simulink model "kaiguangai1108"  (R2016b)
settings: Solver=ode4  StartTime=0.0  StopTime=inf  FixedStep=0.002  RelTol=1e-3  EnableMultiTasking=on
libraries: slrtlib x5
(part 2 of 6)

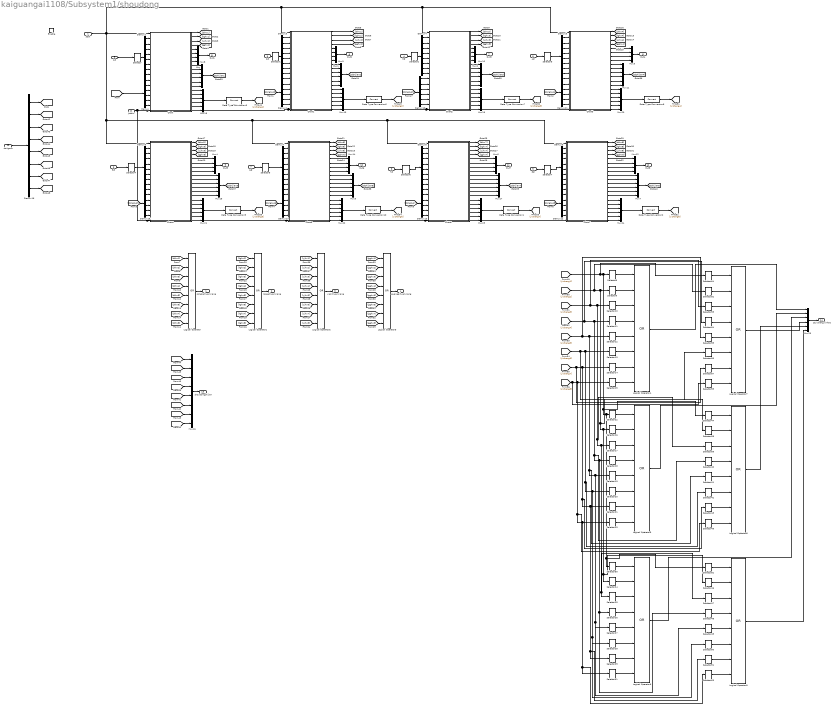
== system kaiguangai1108/Subsystem1/shoudong ==
  start : Inport
  1# : Inport  Port=2
  2# : Inport  Port=3
  3# : Inport  Port=4
  4# : Inport  Port=5
  5# : Inport  Port=6
  6# : Inport  Port=7
  7# : Inport  Port=8
  8# : Inport  Port=9
  dongzuo : Inport  Port=10
  jieshu : Inport  Port=11
  Enable : EnablePort
  Chart : Stateflow chart  TreatAsAtomicUnit=on
  Chart1 : Stateflow chart  TreatAsAtomicUnit=on
  Chart2 : Stateflow chart  TreatAsAtomicUnit=on
  Chart3 : Stateflow chart  TreatAsAtomicUnit=on
  Chart4 : Stateflow chart  TreatAsAtomicUnit=on
  Chart5 : Stateflow chart  TreatAsAtomicUnit=on
  Chart6 : Stateflow chart  TreatAsAtomicUnit=on
  Chart7 : Stateflow chart  TreatAsAtomicUnit=on
  Data Type Conversion{1..2,5..10} (8 alike) : DataTypeConversion
  Demux{,1,10..15} (8 alike) : Demux  Outputs=6
  Demux{2..9,16} (9 alike) : Demux  Outputs=8
  Logical Operator{,1..9} (10 alike) : Logic  Operator=OR  Inputs=8  AllPortsSameDT=off  OutDataTypeStr=boolean
  Mux{,1..4,6,12,14} (8 alike) : Mux
  Mux{5,7..11,13,15,17..25} (17 alike) : Mux  Inputs=6
  Mux16 : Mux  Inputs=8
  Selector{,1..7} (8 alike) : Selector  IndexOptions=Index vector (dialog)  Indices=[1:4 7:10]  OutputSizes=1
  Selector{8..15} (8 alike) : Selector  IndexOptions=Index vector (dialog)  Indices=[1]  OutputSizes=1
  Selector{16..23} (8 alike) : Selector  IndexOptions=Index vector (dialog)  Indices=[2]  OutputSizes=1
  Selector{24..31} (8 alike) : Selector  IndexOptions=Index vector (dialog)  Indices=[3]  OutputSizes=1
  Selector{32..37,54..55} (8 alike) : Selector  IndexOptions=Index vector (dialog)  Indices=[4]  OutputSizes=1
  Selector{38..45} (8 alike) : Selector  IndexOptions=Index vector (dialog)  Indices=[5]  OutputSizes=1
  Selector{46..53} (8 alike) : Selector  IndexOptions=Index vector (dialog)  Indices=[6]  OutputSizes=1
  songkaihuanxiang : Outport
  kaigaihuanxiang : Outport  Port=2
  yajinhuanxiang : Outport  Port=3
  guangaihuanxiang : Outport  Port=4
  Out1 : Outport  Port=5
  Out2 : Outport  Port=6
  Out3 : Outport  Port=7
  Out4 : Outport  Port=8
  Out5 : Outport  Port=9
  Out6 : Outport  Port=10
  Out7 : Outport  Port=11
  Out8 : Outport  Port=12
  shoudongshijian : Outport  Port=13
  sdyichangxinhao : Outport  Port=14
  wires:
  Demux14/2 -> Chart5/11(kaigai)
  Demux14/3 -> Chart5/12(suoding)
  Demux14/1 -> Chart5/10(songkai)
  Demux14/4 -> Chart5/13(jiesuo)
  Demux14/5 -> Chart5/14(guangai)
  Demux14/6 -> Chart5/15(yajin)
  Demux11/4 -> Chart3/13(jiesuo)
  Demux11/5 -> Chart3/14(guangai)
  Demux11/6 -> Chart3/15(yajin)
  Demux13/1 -> Chart6/10(songkai)
  Demux13/2 -> Chart6/11(kaigai)
  Demux13/3 -> Chart6/12(suoding)
  Demux13/4 -> Chart6/13(jiesuo)
  Demux13/5 -> Chart6/14(guangai)
  Demux13/6 -> Chart6/15(yajin)
  Demux9/5 -> Chart7/6(sddw)
  Demux9/6 -> Chart7/7(jsdw)
  Demux9/4 -> Chart7/5(ggdw2)
  Demux9/1 -> Chart7/2(kgdw1)
  Demux9/3 -> Chart7/4(ggdw1)
  Demux9/2 -> Chart7/3(kgdw2)
  Demux9/7 -> Chart7/8(yjdw)
  8#/1 -> Selector7/1
  Demux9/8 -> Chart7/9(skdw)
  Demux11/1 -> Chart3/10(songkai)
  Demux11/2 -> Chart3/11(kaigai)
  Demux11/3 -> Chart3/12(suoding)
  Demux1/1 -> Chart1/10(songkai)
  Demux1/3 -> Chart1/12(suoding)
  Demux1/2 -> Chart1/11(kaigai)
  Demux1/4 -> Chart1/13(jiesuo)
  Demux1/5 -> Chart1/14(guangai)
  Demux1/6 -> Chart1/15(yajin)
  Demux10/1 -> Chart2/10(songkai)
  Demux10/2 -> Chart2/11(kaigai)
  Demux10/4 -> Chart2/13(jiesuo)
  Demux10/5 -> Chart2/14(guangai)
  Demux10/6 -> Chart2/15(yajin)
  Demux10/3 -> Chart2/12(suoding)
  Demux6/1 -> Chart4/2(kgdw1)
  Demux6/2 -> Chart4/3(kgdw2)
  Demux6/3 -> Chart4/4(ggdw1)
  Demux6/4 -> Chart4/5(ggdw2)
  Demux6/5 -> Chart4/6(sddw)
  Demux6/6 -> Chart4/7(jsdw)
  Demux6/7 -> Chart4/8(yjdw)
  Demux6/8 -> Chart4/9(skdw)
  Demux2/3 -> Chart/4(ggdw1)
  Demux8/3 -> Chart6/4(ggdw1)
  Demux8/4 -> Chart6/5(ggdw2)
  Demux8/1 -> Chart6/2(kgdw1)
  Demux8/2 -> Chart6/3(kgdw2)
  Demux8/5 -> Chart6/6(sddw)
  Demux12/1 -> Chart7/10(songkai)
  Demux12/2 -> Chart7/11(kaigai)
  Demux8/8 -> Chart6/9(skdw)
  Demux8/7 -> Chart6/8(yjdw)
  Demux12/3 -> Chart7/12(suoding)
  Demux8/6 -> Chart6/7(jsdw)
  Demux12/6 -> Chart7/15(yajin)
  Demux12/5 -> Chart7/14(guangai)
  Demux12/4 -> Chart7/13(jiesuo)
  Demux15/2 -> Chart4/11(kaigai)
  Demux15/1 -> Chart4/10(songkai)
  Demux5/4 -> Chart3/5(ggdw2)
  Demux5/6 -> Chart3/7(jsdw)
  Demux5/3 -> Chart3/4(ggdw1)
  Demux5/7 -> Chart3/8(yjdw)
  Demux5/5 -> Chart3/6(sddw)
  Demux5/2 -> Chart3/3(kgdw2)
  Demux15/3 -> Chart4/12(suoding)
  Demux5/1 -> Chart3/2(kgdw1)
  4#/1 -> Selector3/1
  Demux5/8 -> Chart3/9(skdw)
  Demux2/7 -> Chart/8(yjdw)
  Demux15/4 -> Chart4/13(jiesuo)
  Demux15/5 -> Chart4/14(guangai)
  Demux15/6 -> Chart4/15(yajin)
  Demux/4 -> Chart/13(jiesuo)
  Demux/5 -> Chart/14(guangai)
  Demux/6 -> Chart/15(yajin)
  Demux2/2 -> Chart/3(kgdw2)
  Demux2/1 -> Chart/2(kgdw1)
  Demux4/2 -> Chart2/3(kgdw2)
  Demux4/3 -> Chart2/4(ggdw1)
  Demux4/4 -> Chart2/5(ggdw2)
  Demux4/5 -> Chart2/6(sddw)
  Demux4/1 -> Chart2/2(kgdw1)
  Demux4/7 -> Chart2/8(yjdw)
  Demux4/6 -> Chart2/7(jsdw)
  Demux4/8 -> Chart2/9(skdw)
  Demux2/4 -> Chart/5(ggdw2)
  Demux2/5 -> Chart/6(sddw)
  Demux2/6 -> Chart/7(jsdw)
  Demux3/2 -> Chart1/3(kgdw2)
  Demux3/3 -> Chart1/4(ggdw1)
  Demux3/4 -> Chart1/5(ggdw2)
  Demux3/6 -> Chart1/7(jsdw)
  Demux3/7 -> Chart1/8(yjdw)
  Demux3/8 -> Chart1/9(skdw)
  Demux2/8 -> Chart/9(skdw)
  Demux3/5 -> Chart1/6(sddw)
  Demux3/1 -> Chart1/2(kgdw1)
  Demux/1 -> Chart/10(songkai)
  Demux/2 -> Chart/11(kaigai)
  Demux/3 -> Chart/12(suoding)
  Demux7/2 -> Chart5/3(kgdw2)
  Demux7/5 -> Chart5/6(sddw)
  Demux7/3 -> Chart5/4(ggdw1)
  Demux7/1 -> Chart5/2(kgdw1)
  Demux7/8 -> Chart5/9(skdw)
  Demux7/4 -> Chart5/5(ggdw2)
  6#/1 -> Selector5/1
  Demux7/6 -> Chart5/7(jsdw)
  Demux7/7 -> Chart5/8(yjdw)
  5#/1 -> Selector4/1
  7#/1 -> Selector6/1
  [dongzuo2] -> Demux1/1
  [dongzuo3] -> Demux10/1
  [dongzuo4] -> Demux11/1
  [dongzuo5] -> Demux15/1
  [dongzuo6] -> Demux14/1
  [dongzuo7] -> Demux13/1
  [dongzuo8] -> Demux12/1
  Chart/1(skhx) -> [skhx1]
  Chart/2(kghx) -> [kghx1]
  Chart/3(yjhx) -> [yjhx1]
  Chart/4(gghx) -> [gghx1]
  Chart1/1(skhx) -> [skhx2]
  Chart1/2(kghx) -> [kghx2]
  Chart1/3(yjhx) -> [yjhx2]
  Chart1/4(gghx) -> [gghx2]
  Chart2/1(skhx) -> [skhx3]
  Chart2/2(kghx) -> [kghx3]
  Chart2/3(yjhx) -> [yjhx3]
  Chart2/4(gghx) -> [gghx3]
  Chart3/1(skhx) -> [skhx4]
  Chart3/2(kghx) -> [kghx4]
  Chart3/3(yjhx) -> [yjhx4]
  Chart3/4(gghx) -> [gghx4]
  Chart4/1(skhx) -> [skhx5]
  Chart5/1(skhx) -> [skhx6]
  Chart5/2(kghx) -> [kghx6]
  Chart5/4(gghx) -> [gghx6]
  Chart7/1(skhx) -> [skhx8]
  Chart7/2(kghx) -> [kghx8]
  Chart7/3(yjhx) -> [yjhx8]
  Chart7/4(gghx) -> [gghx8]
  [skhx1] -> Logical Operator/1
  [skhx2] -> Logical Operator/2
  [skhx3] -> Logical Operator/3
  [skhx4] -> Logical Operator/4
  [skhx5] -> Logical Operator/5
  [skhx6] -> Logical Operator/6
  [skhx7] -> Logical Operator/7
  [skhx8] -> Logical Operator/8
  Logical Operator/1 -> songkaihuanxiang/1
  [kghx1] -> Logical Operator1/1
  [kghx2] -> Logical Operator1/2
  [kghx3] -> Logical Operator1/3
  [kghx4] -> Logical Operator1/4
  [kghx5] -> Logical Operator1/5
  [kghx6] -> Logical Operator1/6
  [kghx7] -> Logical Operator1/7
  [kghx8] -> Logical Operator1/8
  Logical Operator1/1 -> kaigaihuanxiang/1
  [yjhx1] -> Logical Operator2/1
  [yjhx2] -> Logical Operator2/2
  [yjhx3] -> Logical Operator2/3
  [yjhx4] -> Logical Operator2/4
  [yjhx5] -> Logical Operator2/5
  [yjhx6] -> Logical Operator2/6
  [yjhx7] -> Logical Operator2/7
  [yjhx8] -> Logical Operator2/8
  Logical Operator2/1 -> yajinhuanxiang/1
  [gghx1] -> Logical Operator3/1
  [gghx2] -> Logical Operator3/2
  [gghx3] -> Logical Operator3/3
  [gghx4] -> Logical Operator3/4
  [gghx5] -> Logical Operator3/5
  [gghx6] -> Logical Operator3/6
  [gghx7] -> Logical Operator3/7
  [gghx8] -> Logical Operator3/8
  Logical Operator3/1 -> guangaihuanxiang/1
  Chart/5(kgzhiling1) -> Mux/1
  Chart/6(kgzhiling2) -> Mux/2
  Chart/7(ggzhiling1) -> Mux/3
  Chart/8(ggzhiling2) -> Mux/4
  Chart1/5(kgzhiling1) -> Mux1/1
  Chart1/6(kgzhiling2) -> Mux1/2
  Chart1/7(ggzhiling1) -> Mux1/3
  Chart1/8(ggzhiling2) -> Mux1/4
  Chart2/5(kgzhiling1) -> Mux2/1
  Chart2/6(kgzhiling2) -> Mux2/2
  Chart2/7(ggzhiling1) -> Mux2/3
  Chart2/8(ggzhiling2) -> Mux2/4
  Mux/1 -> Out1/1
  Mux1/1 -> Out2/1
  Mux2/1 -> Out3/1
  Mux4/1 -> Out5/1
  Mux14/1 -> Out6/1
  Chart/9(skt) -> Mux8/1
  Chart/10(kgt) -> Mux8/2
  Chart/11(sdt) -> Mux8/3
  Chart/12(jst) -> Mux8/4
  Chart/13(ggt) -> Mux8/5
  Chart/14(yjt) -> Mux8/6
  Chart1/9(skt) -> Mux9/1
  Chart1/10(kgt) -> Mux9/2
  Chart1/11(sdt) -> Mux9/3
  Chart1/12(jst) -> Mux9/4
  Chart1/13(ggt) -> Mux9/5
  Chart1/14(yjt) -> Mux9/6
  Mux8/1 -> [sdshijian1]
  Mux9/1 -> [sdshijian2]
  Mux17/1 -> [sdshijian7]
  [sdshijian1] -> Mux16/1
  [sdshijian2] -> Mux16/2
  [sdshijian3] -> Mux16/3
  [sdshijian4] -> Mux16/4
  [sdshijian5] -> Mux16/5
  [sdshijian6] -> Mux16/6
  [sdshijian7] -> Mux16/7
  [sdshijian8] -> Mux16/8
  Mux16/1 -> shoudongshijian/1
  Selector/1 -> Demux2/1
  1#/1 -> Selector/1
  2#/1 -> Selector1/1
  Selector1/1 -> Demux3/1
  Selector2/1 -> Demux4/1
  3#/1 -> Selector2/1
  Selector3/1 -> Demux5/1
  Selector4/1 -> Demux6/1
  Selector5/1 -> Demux7/1
  Selector6/1 -> Demux8/1
  Selector7/1 -> Demux9/1
  jieshu/1 -> Chart7/16(jieshu), Chart6/16(jieshu), Chart5/16(jieshu), Chart4/16(jieshu), Chart3/16(jieshu), Chart2/16(jieshu), Chart1/16(jieshu), Chart/16(jieshu)
  Demux16/1 -> [dongzuo1]
  [dongzuo1] -> Demux/1
  Demux16/2 -> [dongzuo2]
  Demux16/3 -> [dongzuo3]
  Demux16/4 -> [dongzuo4]
  Demux16/5 -> [dongzuo5]
  Demux16/6 -> [dongzuo6]
  Demux16/7 -> [dongzuo7]
  Demux16/8 -> [dongzuo8]
  dongzuo/1 -> Demux16/1
  Chart2/14(yjt) -> Mux10/6
  Chart2/13(ggt) -> Mux10/5
  Chart2/12(jst) -> Mux10/4
  Chart2/11(sdt) -> Mux10/3
  Chart2/10(kgt) -> Mux10/2
  Chart2/9(skt) -> Mux10/1
  Mux10/1 -> [sdshijian3]
  Chart3/8(ggzhiling2) -> Mux3/4
  Chart3/7(ggzhiling1) -> Mux3/3
  Chart3/6(kgzhiling2) -> Mux3/2
  Chart3/5(kgzhiling1) -> Mux3/1
  Mux3/1 -> Out4/1
  Chart3/9(skt) -> Mux11/1
  Chart3/10(kgt) -> Mux11/2
  Chart3/11(sdt) -> Mux11/3
  Chart3/12(jst) -> Mux11/4
  Chart3/13(ggt) -> Mux11/5
  Chart3/14(yjt) -> Mux11/6
  Mux11/1 -> [sdshijian4]
  Chart4/2(kghx) -> [kghx5]
  Chart4/3(yjhx) -> [yjhx5]
  Chart4/4(gghx) -> [gghx5]
  Chart4/5(kgzhiling1) -> Mux4/1
  Chart4/6(kgzhiling2) -> Mux4/2
  Chart4/7(ggzhiling1) -> Mux4/3
  Chart4/8(ggzhiling2) -> Mux4/4
  Chart4/9(skt) -> Mux15/1
  Chart4/10(kgt) -> Mux15/2
  Chart4/11(sdt) -> Mux15/3
  Chart4/12(jst) -> Mux15/4
  Chart4/13(ggt) -> Mux15/5
  Chart4/14(yjt) -> Mux15/6
  Mux15/1 -> [sdshijian5]
  Chart5/3(yjhx) -> [yjhx6]
  Chart5/5(kgzhiling1) -> Mux14/1
  Chart5/6(kgzhiling2) -> Mux14/2
  Chart5/7(ggzhiling1) -> Mux14/3
  Chart5/8(ggzhiling2) -> Mux14/4
  Chart5/9(skt) -> Mux5/1
  Chart5/10(kgt) -> Mux5/2
  Chart5/11(sdt) -> Mux5/3
  Chart5/12(jst) -> Mux5/4
  Chart5/13(ggt) -> Mux5/5
  Chart5/14(yjt) -> Mux5/6
  Mux5/1 -> [sdshijian6]
  Chart6/1(skhx) -> [skhx7]
  Chart6/2(kghx) -> [kghx7]
  Chart6/3(yjhx) -> [yjhx7]
  Chart6/4(gghx) -> [gghx7]
  Chart6/8(ggzhiling2) -> Mux6/4
  Chart6/7(ggzhiling1) -> Mux6/3
  Chart6/6(kgzhiling2) -> Mux6/2
  Chart6/5(kgzhiling1) -> Mux6/1
  Mux6/1 -> Out7/1
  Chart6/10(kgt) -> Mux17/2
  Chart6/11(sdt) -> Mux17/3
  Chart6/12(jst) -> Mux17/4
  Chart6/13(ggt) -> Mux17/5
  Chart6/14(yjt) -> Mux17/6
  Chart6/9(skt) -> Mux17/1
  Mux7/1 -> [sdshijian8]
  Chart7/8(ggzhiling2) -> Mux12/4
  Chart7/7(ggzhiling1) -> Mux12/3
  Chart7/6(kgzhiling2) -> Mux12/2
  Chart7/5(kgzhiling1) -> Mux12/1
  Mux12/1 -> Out8/1
  Chart7/10(kgt) -> Mux7/2
  Chart7/11(sdt) -> Mux7/3
  Chart7/12(jst) -> Mux7/4
  Chart7/13(ggt) -> Mux7/5
  Chart7/14(yjt) -> Mux7/6
  Chart7/9(skt) -> Mux7/1
  Chart1/15(skyichang) -> Mux13/1
  Chart1/16(kgyichang) -> Mux13/2
  Chart1/17(sdyichang) -> Mux13/3
  Chart1/18(jsyichang) -> Mux13/4
  Chart1/19(ggyichang) -> Mux13/5
  Chart1/20(yjyichang) -> Mux13/6
  Chart/15(skyichang) -> Mux18/1
  Chart/16(kgyichang) -> Mux18/2
  Chart/17(sdyichang) -> Mux18/3
  Chart/18(jsyichang) -> Mux18/4
  Chart/19(ggyichang) -> Mux18/5
  Chart/20(yjyichang) -> Mux18/6
  Chart2/15(skyichang) -> Mux19/1
  Chart2/16(kgyichang) -> Mux19/2
  Chart2/17(sdyichang) -> Mux19/3
  Chart2/18(jsyichang) -> Mux19/4
  Chart2/19(ggyichang) -> Mux19/5
  Chart2/20(yjyichang) -> Mux19/6
  Chart3/15(skyichang) -> Mux20/1
  Chart3/16(kgyichang) -> Mux20/2
  Chart3/17(sdyichang) -> Mux20/3
  Chart3/18(jsyichang) -> Mux20/4
  Chart3/19(ggyichang) -> Mux20/5
  Chart3/20(yjyichang) -> Mux20/6
  Chart4/15(skyichang) -> Mux21/1
  Chart4/16(kgyichang) -> Mux21/2
  Chart4/17(sdyichang) -> Mux21/3
  Chart4/18(jsyichang) -> Mux21/4
  Chart4/19(ggyichang) -> Mux21/5
  Chart4/20(yjyichang) -> Mux21/6
  Chart5/15(skyichang) -> Mux22/1
  Chart5/16(kgyichang) -> Mux22/2
  Chart5/17(sdyichang) -> Mux22/3
  Chart5/18(jsyichang) -> Mux22/4
  Chart5/19(ggyichang) -> Mux22/5
  Chart5/20(yjyichang) -> Mux22/6
  Chart6/15(skyichang) -> Mux23/1
  Chart6/16(kgyichang) -> Mux23/2
  Chart6/17(sdyichang) -> Mux23/3
  Chart6/18(jsyichang) -> Mux23/4
  Chart6/19(ggyichang) -> Mux23/5
  Chart6/20(yjyichang) -> Mux23/6
  Chart7/15(skyichang) -> Mux24/1
  Chart7/16(kgyichang) -> Mux24/2
  Chart7/17(sdyichang) -> Mux24/3
  Chart7/18(jsyichang) -> Mux24/4
  Chart7/19(ggyichang) -> Mux24/5
  Chart7/20(yjyichang) -> Mux24/6
  Mux18/1 -> Data Type Conversion5/1
  Data Type Conversion5/1 -> [yichang1]
  Mux13/1 -> Data Type Conversion6/1
  Data Type Conversion6/1 -> [yichang2]
  Mux19/1 -> Data Type Conversion7/1
  Data Type Conversion7/1 -> [yichang3]
  Mux20/1 -> Data Type Conversion8/1
  Data Type Conversion8/1 -> [yichang4]
  Mux21/1 -> Data Type Conversion9/1
  Data Type Conversion9/1 -> [yichang5]
  Mux22/1 -> Data Type Conversion10/1
  Data Type Conversion10/1 -> [yichang6]
  Mux23/1 -> Data Type Conversion1/1
  Data Type Conversion1/1 -> [yichang7]
  Mux24/1 -> Data Type Conversion2/1
  Data Type Conversion2/1 -> [yichang8]
  start/1 -> Chart/1(start), Chart4/1(start), Chart5/1(start), Chart7/1(start), Chart6/1(start), Chart1/1(start), Chart3/1(start), Chart2/1(start)
  Selector8/1 -> Logical Operator4/1
  Selector9/1 -> Logical Operator4/2
  Selector10/1 -> Logical Operator4/3
  Selector11/1 -> Logical Operator4/4
  Selector12/1 -> Logical Operator4/5
  Selector13/1 -> Logical Operator4/6
  Selector14/1 -> Logical Operator4/7
  Selector15/1 -> Logical Operator4/8
  Selector16/1 -> Logical Operator5/2
  Selector17/1 -> Logical Operator5/3
  Selector18/1 -> Logical Operator5/4
  Selector19/1 -> Logical Operator5/5
  Selector20/1 -> Logical Operator5/6
  Selector21/1 -> Logical Operator5/7
  Selector23/1 -> Logical Operator5/8
  Selector30/1 -> Logical Operator6/1
  Selector24/1 -> Logical Operator6/2
  Selector25/1 -> Logical Operator6/3
  Selector26/1 -> Logical Operator6/4
  Selector27/1 -> Logical Operator6/5
  Selector28/1 -> Logical Operator6/6
  Selector29/1 -> Logical Operator6/7
  Selector31/1 -> Logical Operator6/8
  Selector54/1 -> Logical Operator7/1
  Selector32/1 -> Logical Operator7/2
  Selector33/1 -> Logical Operator7/3
  Selector34/1 -> Logical Operator7/4
  Selector35/1 -> Logical Operator7/5
  Selector36/1 -> Logical Operator7/6
  Selector37/1 -> Logical Operator7/7
  Selector55/1 -> Logical Operator7/8
  Selector22/1 -> Logical Operator5/1
  Selector44/1 -> Logical Operator8/1
  Selector38/1 -> Logical Operator8/2
  Selector39/1 -> Logical Operator8/3
  Selector40/1 -> Logical Operator8/4
  Selector41/1 -> Logical Operator8/5
  Selector42/1 -> Logical Operator8/6
  Selector43/1 -> Logical Operator8/7
  Selector45/1 -> Logical Operator8/8
  [yichang1] -> Selector54/1, Selector44/1, Selector52/1, Selector30/1, Selector22/1, Selector8/1
  [yichang2] -> Selector32/1, Selector38/1, Selector16/1, Selector46/1, Selector24/1, Selector9/1
  [yichang3] -> Selector33/1, Selector39/1, Selector17/1, Selector47/1, Selector25/1, Selector10/1
  [yichang4] -> Selector34/1, Selector40/1, Selector18/1, Selector48/1, Selector26/1, Selector11/1
  [yichang5] -> Selector35/1, Selector41/1, Selector19/1, Selector49/1, Selector27/1, Selector12/1
  [yichang6] -> Selector36/1, Selector42/1, Selector20/1, Selector50/1, Selector28/1, Selector13/1
  [yichang7] -> Selector37/1, Selector43/1, Selector21/1, Selector51/1, Selector29/1, Selector14/1
  [yichang8] -> Selector55/1, Selector45/1, Selector23/1, Selector53/1, Selector31/1, Selector15/1
  Selector52/1 -> Logical Operator9/1
  Selector46/1 -> Logical Operator9/2
  Selector47/1 -> Logical Operator9/3
  Selector48/1 -> Logical Operator9/4
  Selector49/1 -> Logical Operator9/5
  Selector50/1 -> Logical Operator9/6
  Selector51/1 -> Logical Operator9/7
  Selector53/1 -> Logical Operator9/8
  Logical Operator4/1 -> Mux25/1
  Logical Operator5/1 -> Mux25/2
  Logical Operator6/1 -> Mux25/3
  Logical Operator7/1 -> Mux25/4
  Logical Operator8/1 -> Mux25/5
  Logical Operator9/1 -> Mux25/6
  Mux25/1 -> sdyichangxinhao/1

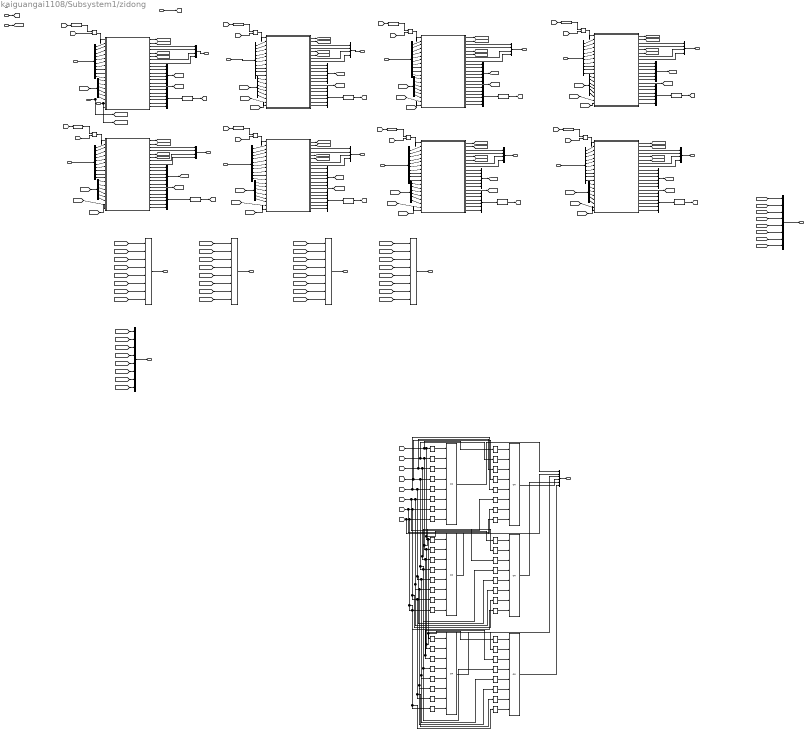
== system kaiguangai1108/Subsystem1/zidong ==
  start : Inport
  In1 : Inport  Port=2
  In2 : Inport  Port=3
  In3 : Inport  Port=4
  In4 : Inport  Port=5
  In5 : Inport  Port=6
  In6 : Inport  Port=7
  In7 : Inport  Port=8
  In8 : Inport  Port=9
  "jiangeshijian " : Inport  Port=10
  shedingcishu : Inport  Port=11
  jieshu : Inport  Port=12
  jinggaixuanze : Inport  Port=13
  Enable : EnablePort
  1# : Stateflow chart  TreatAsAtomicUnit=on
  1#1 : Stateflow chart  TreatAsAtomicUnit=on
  1#2 : Stateflow chart  TreatAsAtomicUnit=on
  1#3 : Stateflow chart  TreatAsAtomicUnit=on
  1#4 : Stateflow chart  TreatAsAtomicUnit=on
  1#5 : Stateflow chart  TreatAsAtomicUnit=on
  1#6 : Stateflow chart  TreatAsAtomicUnit=on
  1#7 : Stateflow chart  TreatAsAtomicUnit=on
  Data Type Conversion1 : DataTypeConversion  OutDataTypeStr=double
  Data Type Conversion{2..8} (7 alike) : DataTypeConversion
  Demux{1..2,4,6,8,12,14,16} (8 alike) : Demux  Outputs=6
  Demux{3,5,7,9..11,13,15} (8 alike) : Demux  Outputs=10
  Logical Operator{,1..3,12..17} (10 alike) : Logic  Operator=OR  Inputs=8  AllPortsSameDT=off  OutDataTypeStr=boolean
  Logical Operator{4..11} (8 alike) : Logic  AllPortsSameDT=off  OutDataTypeStr=boolean
  Mux{,1..7} (8 alike) : Mux
  Mux{8..15,18..26} (17 alike) : Mux  Inputs=6
  Mux16 : Mux  Inputs=8
  Mux17 : Mux  Inputs=8
  Selector{8..15} (8 alike) : Selector  IndexOptions=Index vector (dialog)  Indices=[1]  OutputSizes=1
  Selector{16..23} (8 alike) : Selector  IndexOptions=Index vector (dialog)  Indices=[2]  OutputSizes=1
  Selector{24..31} (8 alike) : Selector  IndexOptions=Index vector (dialog)  Indices=[3]  OutputSizes=1
  Selector{32..37,54..55} (8 alike) : Selector  IndexOptions=Index vector (dialog)  Indices=[4]  OutputSizes=1
  Selector{38..45} (8 alike) : Selector  IndexOptions=Index vector (dialog)  Indices=[5]  OutputSizes=1
  Selector{46..53} (8 alike) : Selector  IndexOptions=Index vector (dialog)  Indices=[6]  OutputSizes=1
  kaigaihuanchong : Selector  InputPortWidth=8  IndexOptions=Index vector (dialog)  Indices=1  OutputSizes=1
  kaigaihuanchong1 : Selector  InputPortWidth=8  IndexOptions=Index vector (dialog)  Indices=2  OutputSizes=1
  kaigaihuanchong2 : Selector  InputPortWidth=8  IndexOptions=Index vector (dialog)  Indices=3  OutputSizes=1
  kaigaihuanchong3 : Selector  InputPortWidth=8  IndexOptions=Index vector (dialog)  Indices=4  OutputSizes=1
  kaigaihuanchong4 : Selector  InputPortWidth=8  IndexOptions=Index vector (dialog)  Indices=5  OutputSizes=1
  kaigaihuanchong5 : Selector  InputPortWidth=8  IndexOptions=Index vector (dialog)  Indices=6  OutputSizes=1
  kaigaihuanchong6 : Selector  InputPortWidth=8  IndexOptions=Index vector (dialog)  Indices=7  OutputSizes=1
  kaigaihuanchong7 : Selector  InputPortWidth=8  IndexOptions=Index vector (dialog)  Indices=8  OutputSizes=1
  songkaihuanxiang : Outport
  kaigaihuanxiang : Outport  Port=2
  yajinhuanxiang : Outport  Port=3
  guangaihuanxiang : Outport  Port=4
  Out1 : Outport  Port=5
  Out2 : Outport  Port=6
  Out3 : Outport  Port=7
  Out4 : Outport  Port=8
  Out5 : Outport  Port=9
  Out6 : Outport  Port=10
  Out7 : Outport  Port=11
  Out8 : Outport  Port=12
  "zidongshijian " : Outport  Port=13
  yikaicishu : Outport  Port=14
  zdyichangxinhao : Outport  Port=15
  wires:
  "jiangeshijian "/1 -> [jiangeshijian]
  Demux1/1 -> 1#/12(t1)
  Demux1/2 -> 1#/13(t3)
  Demux1/3 -> 1#/14(t5)
  Demux1/4 -> 1#/15(t7)
  Demux1/5 -> 1#/16(t9)
  [jiangeshijian] -> Demux1/1
  In1/1 -> Demux9/1  "kaigaidaowei1 kaigaidaowei2 guangaidaowei1 guangaidaowei2 kaigaihuanchong guangaihuanchong suodingdaowei jiesuodaowei yajindaowei songkaidaowei"
  start/1 -> [start]
  [start] -> Logical Operator4/2
  Demux2/1 -> 1#1/12(t1)
  Demux2/2 -> 1#1/13(t3)
  Demux2/3 -> 1#1/14(t5)
  Demux2/4 -> 1#1/15(t7)
  Demux2/5 -> 1#1/16(t9)
  [jiangeshijian] -> Demux2/1
  Demux3/1 -> 1#1/2(kgdw1)
  Demux3/2 -> 1#1/3(kgdw2)
  Demux3/3 -> 1#1/4(ggdw1)
  Demux3/4 -> 1#1/5(ggdw2)
  Demux3/5 -> 1#1/6(kghc)
  Demux3/6 -> 1#1/7(gghc)
  Demux3/7 -> 1#1/8(sddw)
  Demux3/8 -> 1#1/9(jsdw)
  Demux3/9 -> 1#1/10(yjdw)
  Demux3/10 -> 1#1/11(skdw)
  In2/1 -> Demux3/1  "kaigaidaowei1 kaigaidaowei2 guangaidaowei1 guangaidaowei2 kaigaihuanchong guangaihuanchong suodingdaowei jiesuodaowei yajindaowei songkaidaowei"
  [jiangeshijian] -> Demux4/1
  In3/1 -> Demux5/1  "kaigaidaowei1 kaigaidaowei2 guangaidaowei1 guangaidaowei2 kaigaihuanchong guangaihuanchong suodingdaowei jiesuodaowei yajindaowei songkaidaowei"
  [jiangeshijian] -> Demux6/1
  In4/1 -> Demux7/1  "kaigaidaowei1 kaigaidaowei2 guangaidaowei1 guangaidaowei2 kaigaihuanchong guangaihuanchong suodingdaowei jiesuodaowei yajindaowei songkaidaowei"
  [jiangeshijian] -> Demux8/1
  In5/1 -> Demux10/1  "kaigaidaowei1 kaigaidaowei2 guangaidaowei1 guangaidaowei2 kaigaihuanchong guangaihuanchong suodingdaowei jiesuodaowei yajindaowei songkaidaowei"
  [jiangeshijian] -> Demux12/1
  In6/1 -> Demux11/1  "kaigaidaowei1 kaigaidaowei2 guangaidaowei1 guangaidaowei2 kaigaihuanchong guangaihuanchong suodingdaowei jiesuodaowei yajindaowei songkaidaowei"
  [jiangeshijian] -> Demux14/1
  In7/1 -> Demux13/1  "kaigaidaowei1 kaigaidaowei2 guangaidaowei1 guangaidaowei2 kaigaihuanchong guangaihuanchong suodingdaowei jiesuodaowei yajindaowei songkaidaowei"
  [jiangeshijian] -> Demux16/1
  In8/1 -> Demux15/1  "kaigaidaowei1 kaigaidaowei2 guangaidaowei1 guangaidaowei2 kaigaihuanchong guangaihuanchong suodingdaowei jiesuodaowei yajindaowei songkaidaowei"
  Demux15/1 -> 1#7/2(kgdw1)
  Demux15/2 -> 1#7/3(kgdw2)
  Demux15/3 -> 1#7/4(ggdw1)
  Demux15/4 -> 1#7/5(ggdw2)
  Demux15/5 -> 1#7/6(kghc)
  Demux15/6 -> 1#7/7(gghc)
  Demux15/7 -> 1#7/8(sddw)
  Demux15/8 -> 1#7/9(jsdw)
  Demux15/9 -> 1#7/10(yjdw)
  Demux15/10 -> 1#7/11(skdw)
  Demux16/1 -> 1#7/12(t1)
  Demux16/2 -> 1#7/13(t3)
  Demux16/3 -> 1#7/14(t5)
  Demux16/4 -> 1#7/15(t7)
  Demux16/5 -> 1#7/16(t9)
  Demux13/1 -> 1#6/2(kgdw1)
  Demux13/2 -> 1#6/3(kgdw2)
  Demux13/3 -> 1#6/4(ggdw1)
  Demux13/4 -> 1#6/5(ggdw2)
  Demux13/5 -> 1#6/6(kghc)
  Demux13/6 -> 1#6/7(gghc)
  Demux13/7 -> 1#6/8(sddw)
  Demux13/8 -> 1#6/9(jsdw)
  Demux13/9 -> 1#6/10(yjdw)
  Demux13/10 -> 1#6/11(skdw)
  Demux14/1 -> 1#6/12(t1)
  Demux14/2 -> 1#6/13(t3)
  Demux14/3 -> 1#6/14(t5)
  Demux14/4 -> 1#6/15(t7)
  Demux14/5 -> 1#6/16(t9)
  Demux11/1 -> 1#5/2(kgdw1)
  Demux11/2 -> 1#5/3(kgdw2)
  Demux11/3 -> 1#5/4(ggdw1)
  Demux11/4 -> 1#5/5(ggdw2)
  Demux11/5 -> 1#5/6(kghc)
  Demux11/6 -> 1#5/7(gghc)
  Demux11/7 -> 1#5/8(sddw)
  Demux11/8 -> 1#5/9(jsdw)
  Demux11/9 -> 1#5/10(yjdw)
  Demux11/10 -> 1#5/11(skdw)
  Demux12/5 -> 1#5/16(t9)
  Demux12/4 -> 1#5/15(t7)
  Demux12/3 -> 1#5/14(t5)
  Demux12/1 -> 1#5/12(t1)
  Demux12/2 -> 1#5/13(t3)
  Demux8/1 -> 1#4/12(t1)
  Demux8/2 -> 1#4/13(t3)
  Demux8/3 -> 1#4/14(t5)
  Demux8/4 -> 1#4/15(t7)
  Demux8/5 -> 1#4/16(t9)
  Demux10/1 -> 1#4/2(kgdw1)
  Demux10/2 -> 1#4/3(kgdw2)
  Demux10/3 -> 1#4/4(ggdw1)
  Demux10/4 -> 1#4/5(ggdw2)
  Demux10/5 -> 1#4/6(kghc)
  Demux10/6 -> 1#4/7(gghc)
  Demux10/7 -> 1#4/8(sddw)
  Demux10/8 -> 1#4/9(jsdw)
  Demux10/9 -> 1#4/10(yjdw)
  Demux10/10 -> 1#4/11(skdw)
  Demux5/1 -> 1#2/2(kgdw1)
  Demux5/2 -> 1#2/3(kgdw2)
  Demux5/3 -> 1#2/4(ggdw1)
  Demux5/4 -> 1#2/5(ggdw2)
  Demux5/5 -> 1#2/6(kghc)
  Demux5/6 -> 1#2/7(gghc)
  Demux5/7 -> 1#2/8(sddw)
  Demux5/8 -> 1#2/9(jsdw)
  Demux5/9 -> 1#2/10(yjdw)
  Demux5/10 -> 1#2/11(skdw)
  Demux4/1 -> 1#2/12(t1)
  Demux4/2 -> 1#2/13(t3)
  Demux4/3 -> 1#2/14(t5)
  Demux4/4 -> 1#2/15(t7)
  Demux4/5 -> 1#2/16(t9)
  Demux7/1 -> 1#3/2(kgdw1)
  Demux7/2 -> 1#3/3(kgdw2)
  Demux7/3 -> 1#3/4(ggdw1)
  Demux7/4 -> 1#3/5(ggdw2)
  Demux7/5 -> 1#3/6(kghc)
  Demux7/6 -> 1#3/7(gghc)
  Demux7/7 -> 1#3/8(sddw)
  Demux7/8 -> 1#3/9(jsdw)
  Demux7/9 -> 1#3/10(yjdw)
  Demux7/10 -> 1#3/11(skdw)
  Demux6/1 -> 1#3/12(t1)
  Demux6/2 -> 1#3/13(t3)
  Demux6/3 -> 1#3/14(t5)
  Demux6/4 -> 1#3/15(t7)
  Demux6/5 -> 1#3/16(t9)
  1#/1(skhx) -> [songkaihuanxiang1]
  1#/2(kghx) -> [kaigaihuanxiang1]
  1#/5(yjhx) -> [yajinhuanxiang1]
  1#/6(gghx) -> [guangaihuanxiang1]
  1#1/1(skhx) -> [songkaihuanxiang2]
  1#1/2(kghx) -> [kaigaihuanxiang2]
  1#1/5(yjhx) -> [yajinhuanxiang2]
  1#1/6(gghx) -> [guangaihuanxiang2]
  1#2/1(skhx) -> [songkaihuanxiang3]
  1#2/2(kghx) -> [kaigaihuanxiang3]
  1#2/5(yjhx) -> [yajinhuanxiang3]
  1#2/6(gghx) -> [guangaihuanxiang3]
  1#4/2(kghx) -> [kaigaihuanxiang5]
  1#4/1(skhx) -> [songkaihuanxiang5]
  1#5/1(skhx) -> [songkaihuanxiang6]
  1#5/2(kghx) -> [kaigaihuanxiang6]
  1#7/1(skhx) -> [songkaihuanxiang8]
  1#7/2(kghx) -> [kaigaihuanxiang8]
  1#6/1(skhx) -> [songkaihuanxiang7]
  1#6/2(kghx) -> [kaigaihuanxiang7]
  1#6/5(yjhx) -> [yajinhuanxiang7]
  1#6/6(gghx) -> [guangaihuanxiang7]
  1#3/1(skhx) -> [songkaihuanxiang4]
  1#3/2(kghx) -> [kaigaihuanxiang4]
  [songkaihuanxiang1] -> Logical Operator/1
  [songkaihuanxiang2] -> Logical Operator/2
  [songkaihuanxiang3] -> Logical Operator/3
  [songkaihuanxiang4] -> Logical Operator/4
  [songkaihuanxiang5] -> Logical Operator/5
  [songkaihuanxiang8] -> Logical Operator/8
  [songkaihuanxiang7] -> Logical Operator/7
  [songkaihuanxiang6] -> Logical Operator/6
  Logical Operator/1 -> songkaihuanxiang/1
  [kaigaihuanxiang1] -> Logical Operator1/1
  [kaigaihuanxiang2] -> Logical Operator1/2
  [kaigaihuanxiang3] -> Logical Operator1/3
  [kaigaihuanxiang4] -> Logical Operator1/4
  [kaigaihuanxiang5] -> Logical Operator1/5
  [kaigaihuanxiang8] -> Logical Operator1/8
  [kaigaihuanxiang7] -> Logical Operator1/7
  [kaigaihuanxiang6] -> Logical Operator1/6
  Logical Operator1/1 -> kaigaihuanxiang/1
  [yajinhuanxiang1] -> Logical Operator2/1
  [yajinhuanxiang2] -> Logical Operator2/2
  [yajinhuanxiang3] -> Logical Operator2/3
  [yajinhuanxiang4] -> Logical Operator2/4
  [yajinhuanxiang5] -> Logical Operator2/5
  [yajinhuanxiang8] -> Logical Operator2/8
  [yajinhuanxiang7] -> Logical Operator2/7
  [yajinhuanxiang6] -> Logical Operator2/6
  Logical Operator2/1 -> yajinhuanxiang/1
  [guangaihuanxiang1] -> Logical Operator3/1
  [guangaihuanxiang2] -> Logical Operator3/2
  [guangaihuanxiang3] -> Logical Operator3/3
  [guangaihuanxiang4] -> Logical Operator3/4
  [guangaihuanxiang5] -> Logical Operator3/5
  [guangaihuanxiang8] -> Logical Operator3/8
  [guangaihuanxiang7] -> Logical Operator3/7
  [guangaihuanxiang6] -> Logical Operator3/6
  Logical Operator3/1 -> guangaihuanxiang/1
  1#/3(kgzhiling1) -> Mux/1
  1#/4(kgzhiling2) -> Mux/2
  1#/7(ggzhiling1) -> Mux/3
  1#/8(ggzhiling2) -> Mux/4
  1#1/7(ggzhiling1) -> Mux1/3
  Mux/1 -> Out1/1
  Mux1/1 -> Out2/1
  Mux2/1 -> Out3/1
  Mux4/1 -> Out5/1
  1#/9(skt) -> Mux8/1
  1#/10(kgt) -> Mux8/2
  1#/11(sdt) -> Mux8/3
  1#/12(jst) -> Mux8/4
  1#/13(ggt) -> Mux8/5
  1#/14(yjt) -> Mux8/6
  Mux8/1 -> [shijian1]
  Mux11/1 -> [shijian4]
  Mux21/1 -> [shijian5]
  [shijian1] -> Mux16/1
  [shijian2] -> Mux16/2
  [shijian3] -> Mux16/3
  [shijian4] -> Mux16/4
  [shijian5] -> Mux16/5
  [shijian6] -> Mux16/6
  [shijian7] -> Mux16/7
  Mux16/1 -> "zidongshijian "/1
  [shedingcishu] -> 1#5/18(shedingcishu)
  [shedingcishu] -> 1#6/18(shedingcishu)
  [shedingcishu] -> 1#7/18(shedingcishu)
  shedingcishu/1 -> 1#/18(shedingcishu), [shedingcishu]
  [shedingcishu] -> 1#4/18(shedingcishu)
  [shedingcishu] -> 1#1/18(shedingcishu)
  [shedingcishu] -> 1#2/18(shedingcishu)
  [shedingcishu] -> 1#3/18(shedingcishu)
  1#/15(yikaicishu) -> [yikaicishu1]
  1#1/15(yikaicishu) -> [yikaicishu2]
  1#2/15(yikaicishu) -> [yikaicishu3]
  [yikaicishu1] -> Mux17/1
  [yikaicishu4] -> Mux17/4
  [yikaicishu8] -> Mux17/8
  [yikaicishu7] -> Mux17/7
  [yikaicishu6] -> Mux17/6
  [yikaicishu5] -> Mux17/5
  [yikaicishu2] -> Mux17/2
  [yikaicishu3] -> Mux17/3
  Mux17/1 -> yikaicishu/1
  jieshu/1 -> 1#/19(jieshu), [jieshu]
  [jieshu] -> 1#1/19(jieshu)
  [jieshu] -> 1#2/19(jieshu)
  [jieshu] -> 1#3/19(jieshu)
  [jieshu] -> 1#7/19(jieshu)
  [jieshu] -> 1#4/19(jieshu)
  [jieshu] -> 1#5/19(jieshu)
  [jieshu] -> 1#6/19(jieshu)
  Logical Operator4/1 -> 1#/1(start)
  [start] -> Logical Operator5/2
  Logical Operator5/1 -> 1#1/1(start)
  [start] -> Logical Operator6/2
  Logical Operator6/1 -> 1#2/1(start)
  [start] -> Logical Operator7/2
  Logical Operator7/1 -> 1#3/1(start)
  [start] -> Logical Operator8/2
  Logical Operator8/1 -> 1#4/1(start)
  [start] -> Logical Operator9/2
  Logical Operator9/1 -> 1#5/1(start)
  [start] -> Logical Operator10/2
  Logical Operator10/1 -> 1#6/1(start)
  [start] -> Logical Operator11/2
  Logical Operator11/1 -> 1#7/1(start)
  Demux1/6 -> 1#/17(t11)
  Demux2/6 -> 1#1/17(t11)
  Demux4/6 -> 1#2/17(t11)
  Demux6/6 -> 1#3/17(t11)
  Demux8/6 -> 1#4/17(t11)
  Demux12/6 -> 1#5/17(t11)
  Demux14/6 -> 1#6/17(t11)
  Demux16/6 -> 1#7/17(t11)
  1#/16(skyichang) -> Mux18/1
  1#/17(kgyichang) -> Mux18/2
  1#/18(sdyichang) -> Mux18/3
  1#/19(jsyichang) -> Mux18/4
  1#/20(ggyichang) -> Mux18/5
  1#/21(yjyichang) -> Mux18/6
  Mux18/1 -> Data Type Conversion1/1
  Data Type Conversion1/1 -> [zdyichang1]
  1#1/3(kgzhiling1) -> Mux1/1
  1#1/4(kgzhiling2) -> Mux1/2
  1#1/8(ggzhiling2) -> Mux1/4
  1#1/9(skt) -> Mux9/1
  1#1/10(kgt) -> Mux9/2
  1#1/11(sdt) -> Mux9/3
  1#1/12(jst) -> Mux9/4
  1#1/13(ggt) -> Mux9/5
  1#1/14(yjt) -> Mux9/6
  Mux9/1 -> [shijian2]
  1#1/16(skyichang) -> Mux19/1
  1#1/17(kgyichang) -> Mux19/2
  1#1/18(sdyichang) -> Mux19/3
  1#1/19(jsyichang) -> Mux19/4
  1#1/20(ggyichang) -> Mux19/5
  1#1/21(yjyichang) -> Mux19/6
  Mux19/1 -> Data Type Conversion2/1
  Data Type Conversion2/1 -> [zdyichang2]
  1#2/3(kgzhiling1) -> Mux2/1
  1#2/4(kgzhiling2) -> Mux2/2
  1#2/7(ggzhiling1) -> Mux2/3
  1#2/8(ggzhiling2) -> Mux2/4
  1#2/9(skt) -> Mux10/1
  1#2/10(kgt) -> Mux10/2
  1#2/11(sdt) -> Mux10/3
  1#2/12(jst) -> Mux10/4
  1#2/13(ggt) -> Mux10/5
  1#2/14(yjt) -> Mux10/6
  Mux10/1 -> [shijian3]
  1#2/16(skyichang) -> Mux20/1
  1#2/17(kgyichang) -> Mux20/2
  1#2/18(sdyichang) -> Mux20/3
  1#2/19(jsyichang) -> Mux20/4
  1#2/20(ggyichang) -> Mux20/5
  1#2/21(yjyichang) -> Mux20/6
  Mux20/1 -> Data Type Conversion3/1
  Data Type Conversion3/1 -> [zdyichang3]
  1#3/5(yjhx) -> [yajinhuanxiang4]
  1#3/6(gghx) -> [guangaihuanxiang4]
  Mux3/1 -> Out4/1
  1#3/3(kgzhiling1) -> Mux3/1
  1#3/4(kgzhiling2) -> Mux3/2
  1#3/7(ggzhiling1) -> Mux3/3
  1#3/8(ggzhiling2) -> Mux3/4
  1#4/6(gghx) -> [guangaihuanxiang5]
  1#4/5(yjhx) -> [yajinhuanxiang5]
  1#4/3(kgzhiling1) -> Mux4/1
  1#4/4(kgzhiling2) -> Mux4/2
  1#4/7(ggzhiling1) -> Mux4/3
  1#4/8(ggzhiling2) -> Mux4/4
  1#4/9(skt) -> Mux21/1
  1#4/10(kgt) -> Mux21/2
  1#4/11(sdt) -> Mux21/3
  1#4/12(jst) -> Mux21/4
  1#4/13(ggt) -> Mux21/5
  1#4/14(yjt) -> Mux21/6
  1#4/15(yikaicishu) -> [yikaicishu5]
  1#4/17(kgyichang) -> Mux14/2
  1#4/18(sdyichang) -> Mux14/3
  1#4/19(jsyichang) -> Mux14/4
  1#4/20(ggyichang) -> Mux14/5
  1#4/21(yjyichang) -> Mux14/6
  1#4/16(skyichang) -> Mux14/1
  Mux14/1 -> Data Type Conversion4/1
  Data Type Conversion4/1 -> [zdyichang5]
  1#5/15(yikaicishu) -> [yikaicishu6]
  1#5/5(yjhx) -> [yajinhuanxiang6]
  1#5/6(gghx) -> [guangaihuanxiang6]
  1#5/7(ggzhiling1) -> Mux5/3
  Mux5/1 -> Out6/1
  1#5/3(kgzhiling1) -> Mux5/1
  1#5/4(kgzhiling2) -> Mux5/2
  1#5/8(ggzhiling2) -> Mux5/4
  1#5/9(skt) -> Mux15/1
  1#5/10(kgt) -> Mux15/2
  1#5/11(sdt) -> Mux15/3
  1#5/12(jst) -> Mux15/4
  1#5/13(ggt) -> Mux15/5
  1#5/14(yjt) -> Mux15/6
  Mux15/1 -> [shijian6]
  1#5/16(skyichang) -> Mux22/1
  1#5/17(kgyichang) -> Mux22/2
  1#5/18(sdyichang) -> Mux22/3
  1#5/19(jsyichang) -> Mux22/4
  1#5/20(ggyichang) -> Mux22/5
  1#5/21(yjyichang) -> Mux22/6
  Mux22/1 -> Data Type Conversion5/1
  Data Type Conversion5/1 -> [zdyichang6]
  1#6/7(ggzhiling1) -> Mux6/3
  Mux6/1 -> Out7/1
  1#6/3(kgzhiling1) -> Mux6/1
  1#6/4(kgzhiling2) -> Mux6/2
  1#6/8(ggzhiling2) -> Mux6/4
  1#6/9(skt) -> Mux12/1
  1#6/10(kgt) -> Mux12/2
  1#6/11(sdt) -> Mux12/3
  1#6/12(jst) -> Mux12/4
  1#6/13(ggt) -> Mux12/5
  1#6/14(yjt) -> Mux12/6
  Mux12/1 -> [shijian7]
  1#6/15(yikaicishu) -> [yikaicishu7]
  1#6/16(skyichang) -> Mux23/1
  1#6/17(kgyichang) -> Mux23/2
  1#6/18(sdyichang) -> Mux23/3
  1#6/19(jsyichang) -> Mux23/4
  1#6/20(ggyichang) -> Mux23/5
  1#6/21(yjyichang) -> Mux23/6
  Mux23/1 -> Data Type Conversion6/1
  Data Type Conversion6/1 -> [zdyichang7]
  1#7/5(yjhx) -> [yajinhuanxiang8]
  1#7/6(gghx) -> [guangaihuanxiang8]
  1#7/7(ggzhiling1) -> Mux7/3
  Mux7/1 -> Out8/1
  1#7/3(kgzhiling1) -> Mux7/1
  1#7/4(kgzhiling2) -> Mux7/2
  1#7/8(ggzhiling2) -> Mux7/4
  1#7/9(skt) -> Mux13/1
  1#7/10(kgt) -> Mux13/2
  1#7/11(sdt) -> Mux13/3
  1#7/12(jst) -> Mux13/4
  1#7/13(ggt) -> Mux13/5
  1#7/14(yjt) -> Mux13/6
  Mux13/1 -> [shijian8]
  1#7/15(yikaicishu) -> [yikaicishu8]
  1#7/16(skyichang) -> Mux24/1
  1#7/17(kgyichang) -> Mux24/2
  1#7/18(sdyichang) -> Mux24/3
  1#7/19(jsyichang) -> Mux24/4
  1#7/20(ggyichang) -> Mux24/5
  1#7/21(yjyichang) -> Mux24/6
  Mux24/1 -> Data Type Conversion7/1
  Data Type Conversion7/1 -> [zdyichang8]
  [shijian8] -> Mux16/8
  1#3/15(yikaicishu) -> [yikaicishu4]
  1#3/9(skt) -> Mux11/1
  1#3/10(kgt) -> Mux11/2
  1#3/11(sdt) -> Mux11/3
  1#3/12(jst) -> Mux11/4
  1#3/13(ggt) -> Mux11/5
  1#3/14(yjt) -> Mux11/6
  1#3/16(skyichang) -> Mux25/1
  1#3/17(kgyichang) -> Mux25/2
  1#3/18(sdyichang) -> Mux25/3
  1#3/19(jsyichang) -> Mux25/4
  1#3/20(ggyichang) -> Mux25/5
  1#3/21(yjyichang) -> Mux25/6
  Mux25/1 -> Data Type Conversion8/1
  Data Type Conversion8/1 -> [zdyichang4]
  jinggaixuanze/1 -> [A]
  [A] -> kaigaihuanchong/1
  kaigaihuanchong/1 -> Logical Operator4/1
  [A] -> kaigaihuanchong1/1
  kaigaihuanchong1/1 -> Logical Operator5/1
  [A] -> kaigaihuanchong2/1
  kaigaihuanchong2/1 -> Logical Operator6/1
  [A] -> kaigaihuanchong3/1
  kaigaihuanchong3/1 -> Logical Operator7/1
  [A] -> kaigaihuanchong4/1
  kaigaihuanchong4/1 -> Logical Operator8/1
  [A] -> kaigaihuanchong5/1
  kaigaihuanchong5/1 -> Logical Operator9/1
  [A] -> kaigaihuanchong6/1
  kaigaihuanchong6/1 -> Logical Operator10/1
  [A] -> kaigaihuanchong7/1
  kaigaihuanchong7/1 -> Logical Operator11/1
  Selector8/1 -> Logical Operator12/1
  Selector9/1 -> Logical Operator12/2
  Selector10/1 -> Logical Operator12/3
  Selector11/1 -> Logical Operator12/4
  Selector12/1 -> Logical Operator12/5
  Selector13/1 -> Logical Operator12/6
  Selector14/1 -> Logical Operator12/7
  Selector15/1 -> Logical Operator12/8
  Selector16/1 -> Logical Operator13/2
  Selector17/1 -> Logical Operator13/3
  Selector18/1 -> Logical Operator13/4
  Selector19/1 -> Logical Operator13/5
  Selector20/1 -> Logical Operator13/6
  Selector21/1 -> Logical Operator13/7
  Selector23/1 -> Logical Operator13/8
  Selector30/1 -> Logical Operator14/1
  Selector24/1 -> Logical Operator14/2
  Selector25/1 -> Logical Operator14/3
  Selector26/1 -> Logical Operator14/4
  Selector27/1 -> Logical Operator14/5
  Selector28/1 -> Logical Operator14/6
  Selector29/1 -> Logical Operator14/7
  Selector31/1 -> Logical Operator14/8
  Selector54/1 -> Logical Operator15/1
  Selector32/1 -> Logical Operator15/2
  Selector33/1 -> Logical Operator15/3
  Selector34/1 -> Logical Operator15/4
  Selector35/1 -> Logical Operator15/5
  Selector36/1 -> Logical Operator15/6
  Selector37/1 -> Logical Operator15/7
  Selector55/1 -> Logical Operator15/8
  Selector22/1 -> Logical Operator13/1
  Selector44/1 -> Logical Operator16/1
  Selector38/1 -> Logical Operator16/2
  Selector39/1 -> Logical Operator16/3
  Selector40/1 -> Logical Operator16/4
  Selector41/1 -> Logical Operator16/5
  Selector42/1 -> Logical Operator16/6
  Selector43/1 -> Logical Operator16/7
  Selector45/1 -> Logical Operator16/8
  [zdyichang1] -> Selector54/1, Selector44/1, Selector52/1, Selector30/1, Selector22/1, Selector8/1
  [zdyichang2] -> Selector32/1, Selector38/1, Selector16/1, Selector46/1, Selector24/1, Selector9/1
  [zdyichang3] -> Selector33/1, Selector39/1, Selector17/1, Selector47/1, Selector25/1, Selector10/1
  [zdyichang4] -> Selector34/1, Selector40/1, Selector18/1, Selector48/1, Selector26/1, Selector11/1
  [zdyichang5] -> Selector35/1, Selector41/1, Selector19/1, Selector49/1, Selector27/1, Selector12/1
  [zdyichang6] -> Selector36/1, Selector42/1, Selector20/1, Selector50/1, Selector28/1, Selector13/1
  [zdyichang7] -> Selector37/1, Selector43/1, Selector21/1, Selector51/1, Selector29/1, Selector14/1
  [zdyichang8] -> Selector55/1, Selector45/1, Selector23/1, Selector53/1, Selector31/1, Selector15/1
  Selector52/1 -> Logical Operator17/1
  Selector46/1 -> Logical Operator17/2
  Selector47/1 -> Logical Operator17/3
  Selector48/1 -> Logical Operator17/4
  Selector49/1 -> Logical Operator17/5
  Selector50/1 -> Logical Operator17/6
  Selector51/1 -> Logical Operator17/7
  Selector53/1 -> Logical Operator17/8
  Logical Operator12/1 -> Mux26/1
  Logical Operator13/1 -> Mux26/2
  Logical Operator14/1 -> Mux26/3
  Logical Operator15/1 -> Mux26/4
  Logical Operator16/1 -> Mux26/5
  Logical Operator17/1 -> Mux26/6
  Mux26/1 -> zdyichangxinhao/1
  Demux9/1 -> 1#/2(kgdw1)
  Demux9/2 -> 1#/3(kgdw2)
  Demux9/3 -> 1#/4(ggdw1)
  Demux9/10 -> 1#/11(skdw)
  Demux9/9 -> 1#/10(yjdw)
  Demux9/8 -> 1#/9(jsdw)
  Demux9/7 -> 1#/8(sddw)
  Demux9/6 -> 1#/7(gghc)
  Demux9/5 -> 1#/6(kghc)
  Demux9/4 -> 1#/5(ggdw2)

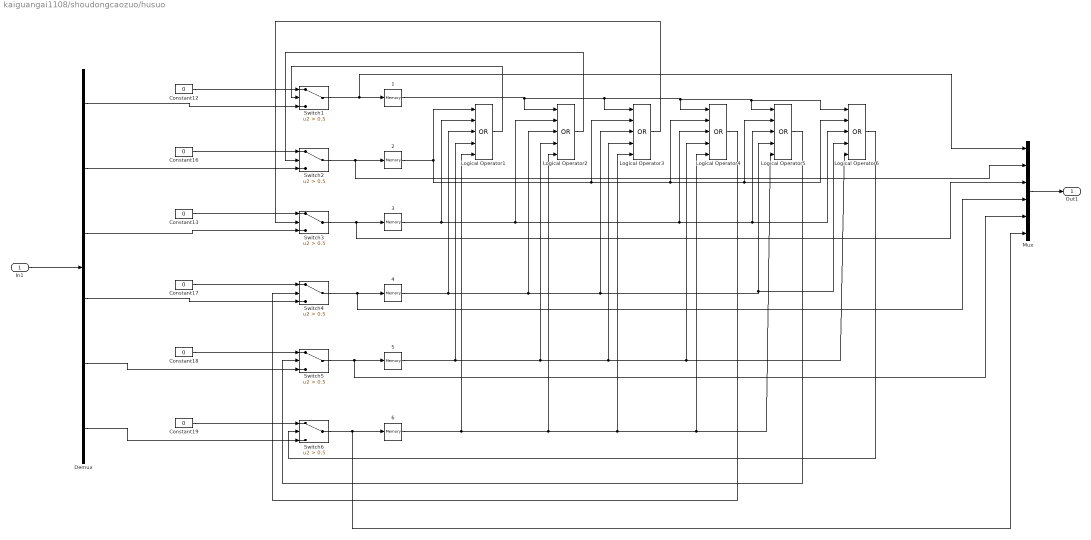
== system kaiguangai1108/shoudongcaozuo/husuo ==
  In1 : Inport
  {1..6} (6 alike) : Memory
  Constant{12..13,16..19} (6 alike) : Constant  Value=0
  Demux : Demux  Outputs=6
  Logical Operator{1..6} (6 alike) : Logic  Operator=OR  Inputs=5  AllPortsSameDT=off  OutDataTypeStr=boolean
  Mux : Mux  Inputs=6
  Switch{1..6} (6 alike) : Switch  Criteria=u2 > Threshold  Threshold=0.5
  Out1 : Outport
  wires:
  In1/1 -> Demux/1
  Mux/1 -> Out1/1
  Constant16/1 -> Switch2/1
  Constant12/1 -> Switch1/1
  Constant17/1 -> Switch4/1
  Constant13/1 -> Switch3/1
  Constant19/1 -> Switch6/1
  Constant18/1 -> Switch5/1
  Switch1/1 -> Mux/1, 1/1
  Switch2/1 -> Mux/2, 2/1
  Switch3/1 -> Mux/3, 3/1
  Switch4/1 -> Mux/4, 4/1
  Switch5/1 -> Mux/5, 5/1
  Switch6/1 -> Mux/6, 6/1
  2/1 -> Logical Operator6/2, Logical Operator5/2, Logical Operator4/2, Logical Operator3/2, Logical Operator1/1
  3/1 -> Logical Operator6/3, Logical Operator5/3, Logical Operator4/3, Logical Operator2/2, Logical Operator1/2
  4/1 -> Logical Operator6/4, Logical Operator5/4, Logical Operator3/3, Logical Operator2/3, Logical Operator1/3
  5/1 -> Logical Operator6/5, Logical Operator4/4, Logical Operator3/4, Logical Operator2/4, Logical Operator1/4
  6/1 -> Logical Operator5/5, Logical Operator4/5, Logical Operator3/5, Logical Operator2/5, Logical Operator1/5
  1/1 -> Logical Operator6/1, Logical Operator5/1, Logical Operator4/1, Logical Operator3/1, Logical Operator2/1
  Logical Operator1/1 -> Switch1/2
  Logical Operator2/1 -> Switch2/2
  Logical Operator3/1 -> Switch3/2
  Logical Operator4/1 -> Switch4/2
  Logical Operator5/1 -> Switch5/2
  Logical Operator6/1 -> Switch6/2
  Demux/2 -> Switch2/3
  Demux/5 -> Switch5/3
  Demux/4 -> Switch4/3
  Demux/1 -> Switch1/3
  Demux/6 -> Switch6/3
  Demux/3 -> Switch3/3

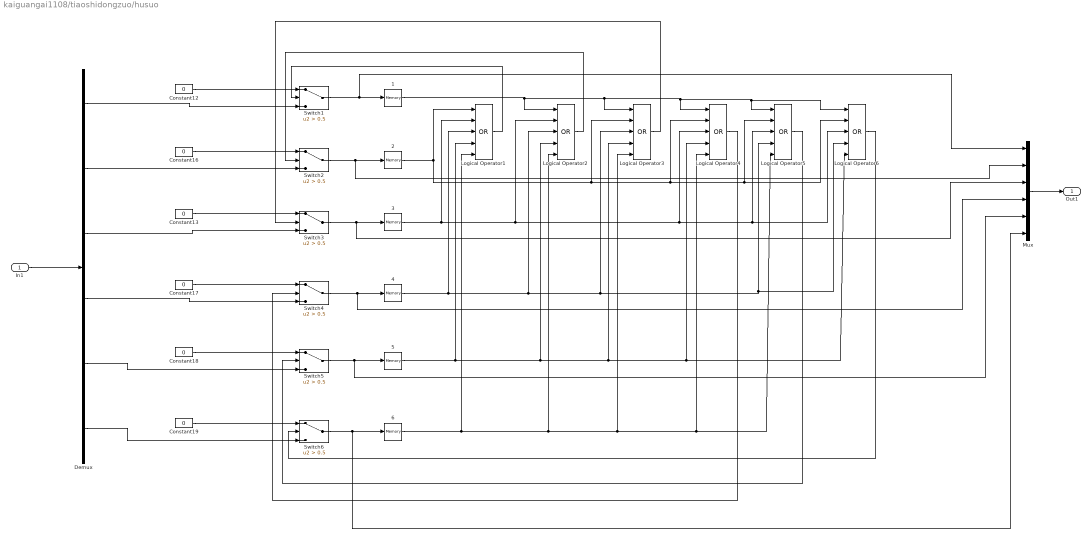
== system kaiguangai1108/tiaoshidongzuo/husuo ==
  In1 : Inport
  {1..6} (6 alike) : Memory
  Constant{12..13,16..19} (6 alike) : Constant  Value=0
  Demux : Demux  Outputs=6
  Logical Operator{1..6} (6 alike) : Logic  Operator=OR  Inputs=5  AllPortsSameDT=off  OutDataTypeStr=boolean
  Mux : Mux  Inputs=6
  Switch{1..6} (6 alike) : Switch  Criteria=u2 > Threshold  Threshold=0.5
  Out1 : Outport
  wires:
  In1/1 -> Demux/1
  Mux/1 -> Out1/1
  Constant16/1 -> Switch2/1
  Constant12/1 -> Switch1/1
  Constant17/1 -> Switch4/1
  Constant13/1 -> Switch3/1
  Constant19/1 -> Switch6/1
  Constant18/1 -> Switch5/1
  Switch1/1 -> Mux/1, 1/1
  Switch2/1 -> Mux/2, 2/1
  Switch3/1 -> Mux/3, 3/1
  Switch4/1 -> Mux/4, 4/1
  Switch5/1 -> Mux/5, 5/1
  Switch6/1 -> Mux/6, 6/1
  2/1 -> Logical Operator6/2, Logical Operator5/2, Logical Operator4/2, Logical Operator3/2, Logical Operator1/1
  3/1 -> Logical Operator6/3, Logical Operator5/3, Logical Operator4/3, Logical Operator2/2, Logical Operator1/2
  4/1 -> Logical Operator6/4, Logical Operator5/4, Logical Operator3/3, Logical Operator2/3, Logical Operator1/3
  5/1 -> Logical Operator6/5, Logical Operator4/4, Logical Operator3/4, Logical Operator2/4, Logical Operator1/4
  6/1 -> Logical Operator5/5, Logical Operator4/5, Logical Operator3/5, Logical Operator2/5, Logical Operator1/5
  1/1 -> Logical Operator6/1, Logical Operator5/1, Logical Operator4/1, Logical Operator3/1, Logical Operator2/1
  Logical Operator1/1 -> Switch1/2
  Logical Operator2/1 -> Switch2/2
  Logical Operator3/1 -> Switch3/2
  Logical Operator4/1 -> Switch4/2
  Logical Operator5/1 -> Switch5/2
  Logical Operator6/1 -> Switch6/2
  Demux/2 -> Switch2/3
  Demux/5 -> Switch5/3
  Demux/4 -> Switch4/3
  Demux/1 -> Switch1/3
  Demux/6 -> Switch6/3
  Demux/3 -> Switch3/3
